simulink model "ESM_TeslaModelS_statKreisfahrt"  (R2020b)
settings: Solver=FixedStepAuto  StartTime=0.0  StopTime=StopTime  FixedStep=SampleTime  RelTol=1e-3
undefined symbols (not defined in the file): ayObs, c_alpha_F, c_alpha_R, c_alpha_rear_mean, DiscIntNeverNeededParam, I_S, init, input_r, m_vehicle, par_TIR, par_VEH, parameter, SelectManeuver, simtime, Single_Track_Model_linear, SingleTrackModel_linear
libraries: pid_lib x5, simulink x3, dspsigops x2, vehicle_model x1
(part 1 of 4)
settings Model: SimulationMode=accelerator  OrderedModelArguments=off  Creator=Johannes  LastModifiedBy=ga69qig
settings DataIOCC: SaveOutput=off  DSMLogging=off  SaveTime=off  ReturnWorkspaceOutputs=off
settings OptimizationCC: EfficientMapNaN2IntZero=off
settings DebuggingCC: ArithmeticOperatorsInVariantConditions=warning
settings HardwareCC: TargetBitPerPointer=64  TargetBitPerSizeT=64  TargetBitPerPtrDiffT=64  TargetLongLongMode=on  TargetIntDivRoundTo=Zero  TargetEndianess=LittleEndian  TargetWordSize=64  TargetHWDeviceType=MATLAB Host  ProdEqTarget=off
settings SFSimCC: SimUseLocalCustomCode=off  CustomCodeUndefinedFunction=UseInterfaceOnly
settings RTWCC: RTWUseLocalCustomCode=off
settings CodeAppCC: MaxIdLength=128
settings GRTTargetCC: TargetLangStandard=C89/C90 (ANSI)  CombineOutputUpdateFcns=off  GRTInterface=on

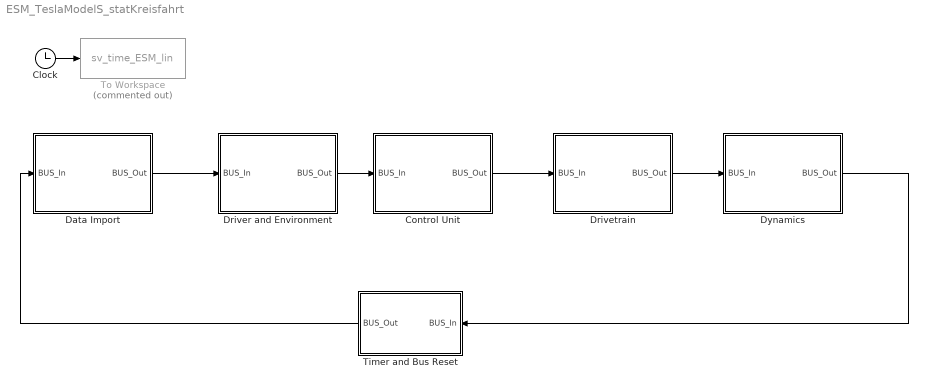
== system ESM_TeslaModelS_statKreisfahrt ==
  Clock : Clock
  Control Unit : Subsystem
      mask help:
      | <Author> Alexander Koch based on Stefan Müller, Stephan Rohr
      | <Date> 03/04/2017
      |
      | <Description>
      | Consist of a Bus In and a Bus Out Block. To Select Signals from the Bus open the Bus In Block, to write signals to the Bus under a certain tab name open the bus out block. For further information, please read the discription of the Bus In and Bus out Block
      |
      | The Block automaticlly disconnects the link to the library block after opening the first time
      |
      | <Parameters>
      | -
      |
      | <Inputs>
      | BUS_In [Bus]
      |
      | <Outputs>
      | Bus_Out [Bus]
      settings: OpenFcn=|
      | set_param(gcb(),'LinkStatus','none')
      | open_system(gcb(),'force')
  Data Import : Subsystem
      mask help:
      | <Author> Alexander Koch based on Stefan Müller, Stephan Rohr
      | <Date> 03/04/2017
      |
      | <Description>
      | Consist of a Bus In and a Bus Out Block. To Select Signals from the Bus open the Bus In Block, to write signals to the Bus under a certain tab name open the bus out block. For further information, please read the discription of the Bus In and Bus out Block
      |
      | The Block automaticlly disconnects the link to the library block after opening the first time
      |
      | <Parameters>
      | -
      |
      | <Inputs>
      | BUS_In [Bus]
      |
      | <Outputs>
      | Bus_Out [Bus]
      settings: OpenFcn=|
      | set_param(gcb(),'LinkStatus','none')
      | open_system(gcb(),'force')
  Driver and Environment : Subsystem
      mask help:
      | <Author> Alexander Koch based on Stefan Müller, Stephan Rohr
      | <Date> 03/04/2017
      |
      | <Description>
      | Consist of a Bus In and a Bus Out Block. To Select Signals from the Bus open the Bus In Block, to write signals to the Bus under a certain tab name open the bus out block. For further information, please read the discription of the Bus In and Bus out Block
      |
      | The Block automaticlly disconnects the link to the library block after opening the first time
      |
      | <Parameters>
      | -
      |
      | <Inputs>
      | BUS_In [Bus]
      |
      | <Outputs>
      | Bus_Out [Bus]
      settings: OpenFcn=|
      | set_param(gcb(),'LinkStatus','none')
      | open_system(gcb(),'force')
  Drivetrain : Subsystem
      mask help:
      | <Author> Alexander Koch based on Stefan Müller, Stephan Rohr
      | <Date> 03/04/2017
      |
      | <Description>
      | Consist of a Bus In and a Bus Out Block. To Select Signals from the Bus open the Bus In Block, to write signals to the Bus under a certain tab name open the bus out block. For further information, please read the discription of the Bus In and Bus out Block
      |
      | The Block automaticlly disconnects the link to the library block after opening the first time
      |
      | <Parameters>
      | -
      |
      | <Inputs>
      | BUS_In [Bus]
      |
      | <Outputs>
      | Bus_Out [Bus]
      settings: OpenFcn=|
      | set_param(gcb(),'LinkStatus','none')
      | open_system(gcb(),'force')
  Dynamics : Subsystem
      mask help:
      | <Author> Alexander Koch based on Stefan Müller, Stephan Rohr
      | <Date> 03/04/2017
      |
      | <Description>
      | Consist of a Bus In and a Bus Out Block. To Select Signals from the Bus open the Bus In Block, to write signals to the Bus under a certain tab name open the bus out block. For further information, please read the discription of the Bus In and Bus out Block
      |
      | The Block automaticlly disconnects the link to the library block after opening the first time
      |
      | <Parameters>
      | -
      |
      | <Inputs>
      | BUS_In [Bus]
      |
      | <Outputs>
      | Bus_Out [Bus]
      settings: OpenFcn=|
      | set_param(gcb(),'LinkStatus','none')
      | open_system(gcb(),'force')
  Timer and Bus Reset : Subsystem
      mask help:
      | <Author> Alexander Koch based on Stefan Müller, Stephan Rohr
      | <Date> 03/04/2017
      |
      | <Description>
      | Initiate a new timestep and creates the Bus_Old with all data of the last time step
      settings: OpenFcn=|
      | set_param(gcb(),'LinkStatus','none')
      | open_system(gcb(),'mask')
      mask DialogControl RefreshBus Prompt: Refresh Bus
      mask DialogControl RefreshBus Callback: TimerandBusResetRefreshBus()
  To Workspace : ToWorkspace  Commented=on  VariableName=sv_time_ESM_lin  SampleTime=-1
      settings: Decimation=savedec  Save2DSignal=2-D array (concatenate along first dimension)
  wires:
  Driver and Environment/1(BUS_Out) -> Control Unit/1(BUS_In)
  Control Unit/1(BUS_Out) -> Drivetrain/1(BUS_In)
  Data Import/1(BUS_Out) -> Driver and Environment/1(BUS_In)
  Drivetrain/1(BUS_Out) -> Dynamics/1(BUS_In)
  Dynamics/1(BUS_Out) -> Timer and Bus Reset/1(BUS_In)
  Timer and Bus Reset/1(BUS_Out) -> Data Import/1(BUS_In)
  Clock/1 -> To Workspace/1

== system ESM_TeslaModelS_statKreisfahrt/Control Unit ==
  BUS_In : Inport
  BUS IN : Subsystem
      mask help:
      | <Author> Alexander Koch, Benedikt Danquah based on Stefan Müller [1], Stephan Rohr [2]  </Author>
      |
      | <Date> 02/05/2017</Date>
      |
      | <Description>
      | Automated BUS IN Block for the Bus System. After the Bus In is connected and receives signals it is possible to choose the required signals by clicking on the block. After choosing the signals it is possible to push the Refresh button. This button builds the required amount of outputs, connects the Bus Selector and the Outputs and rename all the outputs with the corresponding signal name. The Block automaticlly disconnects the link to the library block after opening the first time
      | </Description>
      mask init:
      | BusInInitFct()
      settings: OpenFcn=|
      | set_param(gcb(),'LinkStatus','none')
      | open_system(gcb(),'mask')
      | open_system(strcat(gcb(),'/Bus Selector'),'Parameter')
      mask Help:
      | <Parameters>
      | -
      | </Parameters>
      | 
      | <Inputs>
      | Bus [Bus]
      | </Inputs>
      | 
      | <Outputs>
      | Bus [Bus]
      | SignalName[-]
      | </Outputs>
      | 
      | <Sources>
      | [1] S. Mueller, S. Rohr, W. Schmid, and M. Lienkamp, “Analysing the Influence of Driver Behaviour and Tuning Measures on Battery Aging and Residual Value of Electric Vehicles,” in Proc. EVS30 Symposium, Stuttgart, 2017, pp. 1–12.
      | [2] S. Rohr, “Technisch-wirtschaftliche Analyse des Zweitnutzungs- potentials von Lithium-Ionen-Traktionsbatterien,” Dissertation, Institute of Automotive Technology, Technical University Munich, Munich, 2018.
      | </Sources>
      mask DialogControl Container3 Prompt: Documentation:
      mask DialogControl Control3 Prompt: %<MaskHelp>
      mask DialogControl ParameterGroupVar Prompt: Refresh
      mask DialogControl RefreshOutputs Prompt: Refresh all Output Names
      mask DialogControl RefreshOutputs Callback: BusInInitFct()
  BUS OUT : Subsystem  mask{NumberofInputs=4, NameSys='Control Unit'}
      mask prompts: NumberofInputs "Numper of costum inputs"; NameSys "Name of Bus Subsystem"
      mask help:
      | <Author> Alexander Koch, Benedikt Danquah based on Stefan Müller [1], Stephan Rohr [2]  </Author>
      |
      | <Date> 02/05/2017</Date>
      |
      | <Description>
      | Automated BUS Out Block for the Bus System. Allows to enter the Number of costum inputs and the name of the bus system. After entering the parameters the required amout of Inputs are built and connected to the Bus Creator. The signal names that are connected to the inputs In1, ..., InN are automatically adopted at the Bus signal names and can be found in the Bus under the name of the Bus Subsystem. If the signal (line) to the Inport has no name, the name of the previous blocks outport is taken. If this is not possible, the name if the previous block is taken for the Bus signal name.
      |
      | Additional, there are two buttons. The Refresh Input Names refreshes all Input Names. This is required if signal names are changed or signals are connected for the first time. To build a new system or if another Subsystem is added between existing subsystems, the Refresh Bus Selector is required at every subsystem that is calculated after the new subsystem.
      |
      | The Block automaticlly disconnects the link to the library block after opening the first time
      | </Description>
      mask init:
      | BusRefreshInputs()
      settings: OpenFcn=|
      | set_param(gcb(),'LinkStatus','none')
      | open_system(gcb(),'mask')
      mask Help:
      | <Parameters>
      | Number of costum inputs [-]
      | Name of Bus Subsystem ['abc']
      | </Parameters>
      | 
      | <Inputs>
      | Bus [Bus]
      | In1 [ ]
      | </Inputs>
      | 
      | <Outputs>
      | Bus [Bus]
      | </Outputs>
      | 
      | <Sources>
      | [1] S. Mueller, S. Rohr, W. Schmid, and M. Lienkamp, “Analysing the Influence of Driver Behaviour and Tuning Measures on Battery Aging and Residual Value of Electric Vehicles,” in Proc. EVS30 Symposium, Stuttgart, 2017, pp. 1–12.
      | [2] S. Rohr, “Technisch-wirtschaftliche Analyse des Zweitnutzungs- potentials von Lithium-Ionen-Traktionsbatterien,” Dissertation, Institute of Automotive Technology, Technical University Munich, Munich, 2018.
      | </Sources>
      mask DialogControl Container4 Prompt: Documentation:
      mask DialogControl Control4 Prompt: %<MaskHelp>
      mask DialogControl Container3 Prompt: Refresh
      mask DialogControl RefreshInputNames Prompt: Refresh Input Names
      mask DialogControl RefreshInputNames Callback: BusRefreshLineNames()
      mask DialogControl RefreshBusSelector Prompt: Refresh Bus Selector
      mask DialogControl RefreshBusSelector Callback: BusRefreshBusSelector()
  Control Unit Simple : Subsystem  AncestorBlock=Control_Unit_Simple/Control Unit Simple  mask(SB){Brake_Distribution_Front=0.5, MaxBrkTrq=4200, MaxMotorTrqFront=355.7750901796057, MaxMotorTrqRear=355.7750901796057, LocalSampleTime=-1}
      mask prompts: Brake_Distribution_Front "Brake Distribution Front"; MaxBrkTrq "Maximal Braking Torque"; MaxMotorTrqFront "Maximal Motor Torque Front"; MaxMotorTrqRear "Maximal Motor Torque Rear"; LocalSampleTime "Local System Sample-Time [s]"
      mask help:
      | <Author> Alexander Koch, Benedikt Danquah based on Stefan Müller [1], Stephan Rohr [2]  </Author>
      | <Date> 03/04/2017 </Date>
      |
      | <Description>
      | Requires acceleration pedal position, braking pedal position, a brake distribution, the maximal possible braking torque and tha maximal motor torque and calculates a target drive system torque and a target braking torque for front and rear axle. Minimum drive torques is zero.
      | </Description>
      mask init:
      | GlobalSampleTime = CalcGlobalSampleTime(LocalSampleTime);
      mask Help:
      | <Parameters>
      | Brake distribution front [-]
      | 	<Min> 0 </Min>
      | 	<Max> 1 </Max>
      | Maximal braking torque [Nm]
      | Maximal motor torque [Nm]
      | Local System Sample-Time [s]
      | 	<Min> GlobalSampleTime </Min>
      | Global Sample-Time [s]
      | </Parameters>
      | 
      | <Inputs>
      | AccPedalPos [-]
      | 	<Min> 0 </Min>
      | 	<Max> 1 </Max>
      | BrakePedalPos [-]
      | 	<Min>0 </Min>
      | 	<Max> 1 </Max>
      | </Inputs>
      | 
      | <Outputs>
      | TargetDriveTrqFront [Nm]
      | 	<Min> 0 </Min>
      | TargetDriveTrqRear [Nm]
      | 	<Min> 0 </Min>
      | TargetBrakeTrqFrontAxle [Nm]
      | 	<Max> 0 </Max>
      | TargetBrakeTrqRearAxle [Nm]
      | 	<Max> 0 </Max>
      | </Outputs>
      | <Sources>
      | [1] S. Mueller, S. Rohr, W. Schmid, and M. Lienkamp, “Analysing the Influence of Driver Behaviour and Tuning Measures on Battery Aging and Residual Value of Electric Vehicles,” in Proc. EVS30 Symposium, Stuttgart, 2017, pp. 1–12.
      | [2] S. Rohr, “Technisch-wirtschaftliche Analyse des Zweitnutzungs- potentials von Lithium-Ionen-Traktionsbatterien,” Dissertation, Institute of Automotive Technology, Technical University Munich, Munich, 2018.
      | </Sources>
      mask TypeOptions Brake_Distribution_Front: Brake_Distribution_Front/Value
      mask TypeOptions MaxBrkTrq: MaxBrakeTorque/Value
      mask TypeOptions MaxMotorTrqFront: MaxMotorTorque Front/Value
      mask TypeOptions MaxMotorTrqRear: MaxMotorTorque Rear/Value
      mask TypeOptions LocalSampleTime: AccPedalPos [-]/SampleTime | BrakePedalPos [-]/SampleTime
      mask DialogControl Container3 Prompt: Documentation:
      mask DialogControl DescHelpVar Prompt: %<MaskHelp>
      mask DialogControl Container5 Prompt: Sample Time
      mask Display:
      | [picturexpos,pictureypos,picturewidth,pictureheight] = ...
      |     CalcBlockPicturePosition(gcb,1,0.01,0.1,80,120); % calculating picture position depending on Block size and minimum margin size
      | image('Control_Unit_Simple.svg',[picturexpos pictureypos picturewidth pictureheight]) % plot picture to block
  BUS_Out : Outport
  wires:
  BUS_In/1 -> BUS IN/1(BUS_In)
  BUS OUT/1(BUS_OUT) -> BUS_Out/1
  BUS IN/1(BUS) -> BUS OUT/1(BUS)
  BUS IN/2(AccPedalPos [-]) -> Control Unit Simple/1(AccPedalPos [-])
  BUS IN/3(BrakePedalPos [-]) -> Control Unit Simple/2(BrakePedalPos [-])
  Control Unit Simple/3(TargetBrakeTrqFrontAxle [Nm]) -> BUS OUT/4(In3)  "TargetBrakeTrqFrontAxle [Nm]"
  Control Unit Simple/4(TargetBrakeTrqRearAxle [Nm]) -> BUS OUT/5(In4)  "TargetBrakeTrqRearAxle [Nm]"
  Control Unit Simple/2("TargetDriveTrqRear [Nm] ") -> BUS OUT/3(In2)  "TargetDriveTrqRear [Nm]"
  Control Unit Simple/1("TargetDriveTrqFront [Nm] ") -> BUS OUT/2(In1)  "TargetDriveTrqFront [Nm]"

== system ESM_TeslaModelS_statKreisfahrt/Data Import ==
  BUS_In : Inport
  BUS IN : Subsystem
      mask help:
      | <Author> Alexander Koch based on Stefan Müller, Stephan Rohr
      | <Date> 02/05/2017
      |
      | <Description>
      | Automated BUS IN Block for the Bus System. After the Bus In is connected and receives signals it is possible to choose the required signals by clicking on the block. After choosing the signals it is possible to push the Refresh button. This button builds the required amount of outputs, connects the Bus Selector and the Outputs and rename all the outputs with the corresponding signal name.
      |
      | The Block automaticlly disconnects the link to the library block after opening the first time
      |
      | <Parameters>
      | -
      |
      | <Inputs>
      | Bus [Bus]
      |
      | <Outputs>
      | Bus [Bus]
      | SignalName[-]
      mask init:
      | BusInInitFct()
      settings: OpenFcn=|
      | set_param(gcb(),'LinkStatus','none')
      | open_system(gcb(),'mask')
      | open_system(strcat(gcb(),'/Bus Selector'),'Parameter')
      mask DialogControl ParameterGroupVar Prompt: Refresh
      mask DialogControl RefreshOutputs Prompt: Refresh all Output Names
      mask DialogControl RefreshOutputs Callback: BusInInitFct()
  BUS OUT : Subsystem  mask{NumberofInputs=3, NameSys='Data Import'}
      mask prompts: NumberofInputs "Numper of costum inputs"; NameSys "Name of Bus Subsystem"
      mask help:
      | <Author> Alexander Koch based on Stefan Müller, Stephan Rohr
      | <Date> 02/05/2017
      |
      | <Description>
      | Automated BUS Out Block for the Bus System. Allows to enter the Number of costum inputs and the name of the bus system. After entering the parameters the required amout of Inputs are built and connected to the Bus Creator. The signal names that are connected to the inputs In1, ..., InN are automatically adopted at the Bus signal names and can be found in the Bus under the name of the Bus Subsystem. If the signal (line) to the Inport has no name, the name of the previous blocks outport is taken. If this is not possible, the name if the previous block is taken for the Bus signal name.
      |
      | Additional, there are two buttons. The Refresh Input Names refreshes all Input Names. This is required if signal names are changed or signals are connected for the first time. To build a new system or if another Subsystem is added between existing subsystems, the Refresh Bus Selector is required at every subsystem that is calculated after the new subsystem.
      |
      | The Block automaticlly disconnects the link to the library block after opening the first time
      |
      | <Parameters>
      | Number of costum inputs [-]
      | Name of Bus Subsystem ['abc']
      |
      | <Inputs>
      | Bus [Bus]
      | In1 [ ]
      |
      | <Outputs>
      | Bus [Bus]
      mask init:
      | BusRefreshInputs()
      settings: OpenFcn=|
      | set_param(gcb(),'LinkStatus','none')
      | open_system(gcb(),'mask')
      mask DialogControl Container3 Prompt: Refresh
      mask DialogControl RefreshInputNames Prompt: Refresh Input Names
      mask DialogControl RefreshInputNames Callback: BusRefreshLineNames()
      mask DialogControl RefreshBusSelector Prompt: Refresh Bus Selector
      mask DialogControl RefreshBusSelector Callback: BusRefreshBusSelector()
  Constant : Constant  Value=input_r
  From Workspace1 : FromWorkspace  VariableName=v_maneuver
  From Workspace2 : FromWorkspace  VariableName=delta_maneuver
  Gain : Gain  Gain=pi/180
  Terminator : Terminator
  BUS_Out : Outport  VectorParamsAs1DForOutWhenUnconnected=off
  wires:
  BUS_In/1 -> BUS IN/1(BUS_In)
  BUS OUT/1(BUS_OUT) -> BUS_Out/1
  BUS IN/1(BUS) -> BUS OUT/1(BUS)
  BUS IN/2(omega_F [rad/s]) -> Terminator/1
  From Workspace1/1 -> BUS OUT/3(In2)  "Traget_Velocity [m/s]"
  Gain/1 -> BUS OUT/4(In3)  "Target_Steering_Angle [rad]"
  From Workspace2/1 -> Gain/1  "Target_Steering_Angle [Grad]"
  Constant/1 -> BUS OUT/2(In1)  "Target_Radius [m]"

== system ESM_TeslaModelS_statKreisfahrt/Driver and Environment ==
  BUS_In : Inport
  BUS IN : Subsystem
      mask help:
      | <Author> Alexander Koch based on Stefan Müller, Stephan Rohr
      | <Date> 02/05/2017
      |
      | <Description>
      | Automated BUS IN Block for the Bus System. After the Bus In is connected and receives signals it is possible to choose the required signals by clicking on the block. After choosing the signals it is possible to push the Refresh button. This button builds the required amount of outputs, connects the Bus Selector and the Outputs and rename all the outputs with the corresponding signal name.
      |
      | The Block automaticlly disconnects the link to the library block after opening the first time
      |
      | <Parameters>
      | -
      |
      | <Inputs>
      | Bus [Bus]
      |
      | <Outputs>
      | Bus [Bus]
      | SignalName[-]
      mask init:
      | BusInInitFct()
      settings: OpenFcn=|
      | set_param(gcb(),'LinkStatus','none')
      | open_system(gcb(),'mask')
      | open_system(strcat(gcb(),'/Bus Selector'),'Parameter')
      mask DialogControl ParameterGroupVar Prompt: Refresh
      mask DialogControl RefreshOutputs Prompt: Refresh all Output Names
      mask DialogControl RefreshOutputs Callback: BusInInitFct()
  BUS OUT : Subsystem  mask{NumberofInputs=3, NameSys='Driver and Environment'}
      mask prompts: NumberofInputs "Numper of costum inputs"; NameSys "Name of Bus Subsystem"
      mask help:
      | <Author> Alexander Koch based on Stefan Müller, Stephan Rohr
      | <Date> 02/05/2017
      |
      | <Description>
      | Automated BUS Out Block for the Bus System. Allows to enter the Number of costum inputs and the name of the bus system. After entering the parameters the required amout of Inputs are built and connected to the Bus Creator. The signal names that are connected to the inputs In1, ..., InN are automatically adopted at the Bus signal names and can be found in the Bus under the name of the Bus Subsystem. If the signal (line) to the Inport has no name, the name of the previous blocks outport is taken. If this is not possible, the name if the previous block is taken for the Bus signal name.
      |
      | Additional, there are two buttons. The Refresh Input Names refreshes all Input Names. This is required if signal names are changed or signals are connected for the first time. To build a new system or if another Subsystem is added between existing subsystems, the Refresh Bus Selector is required at every subsystem that is calculated after the new subsystem.
      |
      | The Block automaticlly disconnects the link to the library block after opening the first time
      |
      | <Parameters>
      | Number of costum inputs [-]
      | Name of Bus Subsystem ['abc']
      |
      | <Inputs>
      | Bus [Bus]
      | In1 [ ]
      |
      | <Outputs>
      | Bus [Bus]
      mask init:
      | BusRefreshInputs()
      settings: OpenFcn=|
      | set_param(gcb(),'LinkStatus','none')
      | open_system(gcb(),'mask')
      mask DialogControl Container3 Prompt: Refresh
      mask DialogControl RefreshInputNames Prompt: Refresh Input Names
      mask DialogControl RefreshInputNames Callback: BusRefreshLineNames()
      mask DialogControl RefreshBusSelector Prompt: Refresh Bus Selector
      mask DialogControl RefreshBusSelector Callback: BusRefreshBusSelector()
  Lenkradwinkelsprung : Subsystem  TreatAsAtomicUnit=on
  Multiport Switch : MultiPortSwitch  Inputs=5
  Multiport Switch1 : MultiPortSwitch  Inputs=5
  Multiport Switch2 : MultiPortSwitch  Inputs=5
  SelectManeuver : Constant  Value=SelectManeuver
  Sinuslenken : Subsystem  TreatAsAtomicUnit=on
  quasistationare Kreisfahrt : Subsystem  TreatAsAtomicUnit=on
  quasistationare Kreisfahrt mit Lastwechsel Beschleunigung : Subsystem  TreatAsAtomicUnit=on
  quasistationare Kreisfahrt mit Lastwechsel Verzogerung : Subsystem  TreatAsAtomicUnit=on
  BUS_Out : Outport  VectorParamsAs1DForOutWhenUnconnected=off
  wires:
  BUS OUT/1(BUS_OUT) -> BUS_Out/1
  BUS_In/1 -> BUS IN/1(BUS_In)
  Lenkradwinkelsprung/3(BrakePedalPos [-]) -> Multiport Switch2/5
  quasistationare Kreisfahrt/1(delta_h) -> Multiport Switch/2
  BUS IN/7(Target_Steering_Angle [rad]) -> Sinuslenken/3(Target_Steering_Angle [rad])
  Multiport Switch1/1 -> BUS OUT/3(In2)  "AccPedalPos [-]"
  quasistationare Kreisfahrt mit Lastwechsel Verzogerung/3(BrakePedalPos [-]) -> Multiport Switch2/3
  quasistationare Kreisfahrt mit Lastwechsel Verzogerung/1(delta_h) -> Multiport Switch/3  "delta_h"
  Sinuslenken/2(AccPedalPos [-]) -> Multiport Switch1/6
  Sinuslenken/1(delta_h) -> Multiport Switch/6
  BUS IN/3(Traget_Velocity [m/s]) -> quasistationare Kreisfahrt mit Lastwechsel Verzogerung/2(TargetVelocity [m/s]), quasistationare Kreisfahrt mit Lastwechsel Beschleunigung/2(TargetVelocity [m/s]), Lenkradwinkelsprung/2(TargetVelocity [m/s]), Sinuslenken/2(TargetVelocity [m/s]), quasistationare Kreisfahrt/2(TargetVelocity [m/s])
  BUS IN/6(vx [m/s]) -> quasistationare Kreisfahrt mit Lastwechsel Beschleunigung/5(VelocityX [m/s]), quasistationare Kreisfahrt mit Lastwechsel Verzogerung/5(VelocityX [m/s]), quasistationare Kreisfahrt/5(VelocityX [m/s])
  quasistationare Kreisfahrt mit Lastwechsel Verzogerung/2(AccPedalPos [-]) -> Multiport Switch1/3
  quasistationare Kreisfahrt/2(AccPedalPos [-]) -> Multiport Switch1/2
  quasistationare Kreisfahrt/3(BrakePedalPos [-]) -> Multiport Switch2/2
  BUS IN/5(Target_Radius [m]) -> quasistationare Kreisfahrt mit Lastwechsel Beschleunigung/4(TargetRadius [m]), quasistationare Kreisfahrt mit Lastwechsel Verzogerung/4(TargetRadius [m]), quasistationare Kreisfahrt/4(TargetRadius [m])
  Multiport Switch2/1 -> BUS OUT/4(In3)  "BrakePedalPos [-]"
  Lenkradwinkelsprung/1(delta_h) -> Multiport Switch/5
  BUS IN/1(BUS) -> BUS OUT/1(BUS)
  Multiport Switch/1 -> BUS OUT/2(In1)  "delta_h"
  BUS IN/4(ay [m/s^2]) -> quasistationare Kreisfahrt mit Lastwechsel Verzogerung/3(AccelerationY [m/s]), quasistationare Kreisfahrt mit Lastwechsel Beschleunigung/3(AccelerationY [m/s]), quasistationare Kreisfahrt/3(AccelerationY [m/s])
  Sinuslenken/3(BrakePedalPos [-]) -> Multiport Switch2/6
  SelectManeuver/1 -> Multiport Switch/1, Multiport Switch2/1, Multiport Switch1/1
  BUS IN/2(v) -> quasistationare Kreisfahrt mit Lastwechsel Verzogerung/1(Velocity [m/s]), quasistationare Kreisfahrt mit Lastwechsel Beschleunigung/1(Velocity [m/s]), Lenkradwinkelsprung/1(Velocity [m/s]), Sinuslenken/1(Velocity [m/s]), quasistationare Kreisfahrt/1(Velocity [m/s])
  Lenkradwinkelsprung/2(AccPedalPos [-]) -> Multiport Switch1/5
  quasistationare Kreisfahrt mit Lastwechsel Beschleunigung/1(delta_h) -> Multiport Switch/4
  quasistationare Kreisfahrt mit Lastwechsel Beschleunigung/2(AccPedalPos [-]) -> Multiport Switch1/4
  quasistationare Kreisfahrt mit Lastwechsel Beschleunigung/3(BrakePedalPos [-]) -> Multiport Switch2/4

== system ESM_TeslaModelS_statKreisfahrt/Drivetrain ==
  BUS_In : Inport
  Axle Drive Front : Subsystem  AncestorBlock=Axle_Drive/Axle Drive  mask(SB){ratio=9.34, trq_eff=0.9684, LocalSampleTime=-1}
      mask prompts: ratio "Ratio [-]"; trq_eff "Efficiency [-]"; LocalSampleTime "Local System Sample-Time [s]"
      mask help:
      | <Author> Jan Breithaupt </Author>
      | <Date> 05/03/2018 </Date>
      | <Predecessor> Michael Fries </Predecessor>
      |
      | <Description>
      | Calculates torque, rotational speed and moment of inertia acording to the ratio of the axle drive.
      | </Description>
      mask init:
      | GlobalSampleTime = CalcGlobalSampleTime(LocalSampleTime);
      mask Help:
      | <Parameters>
      | Ratio [-]
      | Efficiency [-]
      | Local System Sample-Time [s]
      | 	<Min> GlobalSampleTime </Min>
      | Global Sample-Time [s]
      | </Parameters>
      | 
      | <Inputs>
      | RotSpdWheel [rad/s]
      | GearboxEntranceTrq [Nm]
      | JredIn [kg m^2]
      | </Inputs>
      | 
      | <Outputs>
      | RotSpdGearboxOut [rad/s]
      | WheelMotTrq[Nm]
      | JredOut [kg m^2]
      | </Outputs>
      mask TypeOptions LocalSampleTime: GearboxEntranceTorque [Nm]/SampleTime | RotSpdWheel [rad//s]/SampleTime | JredIn [kg//m^2]/SampleTime
      mask DialogControl Container3 Prompt: Documentation:
      mask DialogControl Control2 Prompt: %<MaskHelp>
      mask DialogControl Container5 Prompt: Sample Time
      mask Display:
      | [picturexpos,pictureypos,picturewidth,pictureheight] = ...
      |     CalcBlockPicturePosition(gcb,1,0.01,0.1,100,100); % calculating picture position depending on Block size and minimum margin size
      | image('Axle_Drive.svg',[picturexpos pictureypos picturewidth pictureheight]); % plot picture to block
  Axle Drive Rear : Subsystem  AncestorBlock=Axle_Drive/Axle Drive  mask(SB){ratio=9.34, trq_eff=0.9684, LocalSampleTime=-1}
      mask prompts: ratio "Ratio [-]"; trq_eff "Efficiency [-]"; LocalSampleTime "Local System Sample-Time [s]"
      mask help:
      | <Author> Jan Breithaupt </Author>
      | <Date> 05/03/2018 </Date>
      | <Predecessor> Michael Fries </Predecessor>
      |
      | <Description>
      | Calculates torque, rotational speed and moment of inertia acording to the ratio of the axle drive.
      | </Description>
      mask init:
      | GlobalSampleTime = CalcGlobalSampleTime(LocalSampleTime);
      mask Help:
      | <Parameters>
      | Ratio [-]
      | Efficiency [-]
      | Local System Sample-Time [s]
      | 	<Min> GlobalSampleTime </Min>
      | Global Sample-Time [s]
      | </Parameters>
      | 
      | <Inputs>
      | RotSpdWheel [rad/s]
      | GearboxEntranceTrq [Nm]
      | JredIn [kg m^2]
      | </Inputs>
      | 
      | <Outputs>
      | RotSpdGearboxOut [rad/s]
      | WheelMotTrq[Nm]
      | JredOut [kg m^2]
      | </Outputs>
      mask TypeOptions LocalSampleTime: GearboxEntranceTorque [Nm]/SampleTime | RotSpdWheel [rad//s]/SampleTime | JredIn [kg//m^2]/SampleTime
      mask DialogControl Container3 Prompt: Documentation:
      mask DialogControl Control2 Prompt: %<MaskHelp>
      mask DialogControl Container5 Prompt: Sample Time
      mask Display:
      | [picturexpos,pictureypos,picturewidth,pictureheight] = ...
      |     CalcBlockPicturePosition(gcb,1,0.01,0.1,100,100); % calculating picture position depending on Block size and minimum margin size
      | image('Axle_Drive.svg',[picturexpos pictureypos picturewidth pictureheight]); % plot picture to block
  BUS IN : Subsystem
      mask help:
      | <Author> Alexander Koch, Benedikt Danquah based on Stefan Müller [1], Stephan Rohr [2]  </Author>
      |
      | <Date> 02/05/2017</Date>
      |
      | <Description>
      | Automated BUS IN Block for the Bus System. After the Bus In is connected and receives signals it is possible to choose the required signals by clicking on the block. After choosing the signals it is possible to push the Refresh button. This button builds the required amount of outputs, connects the Bus Selector and the Outputs and rename all the outputs with the corresponding signal name. The Block automaticlly disconnects the link to the library block after opening the first time
      | </Description>
      mask init:
      | BusInInitFct()
      settings: OpenFcn=|
      | set_param(gcb(),'LinkStatus','none')
      | open_system(gcb(),'mask')
      | open_system(strcat(gcb(),'/Bus Selector'),'Parameter')
      mask Help:
      | <Parameters>
      | -
      | </Parameters>
      | 
      | <Inputs>
      | Bus [Bus]
      | </Inputs>
      | 
      | <Outputs>
      | Bus [Bus]
      | SignalName[-]
      | </Outputs>
      | 
      | <Sources>
      | [1] S. Mueller, S. Rohr, W. Schmid, and M. Lienkamp, “Analysing the Influence of Driver Behaviour and Tuning Measures on Battery Aging and Residual Value of Electric Vehicles,” in Proc. EVS30 Symposium, Stuttgart, 2017, pp. 1–12.
      | [2] S. Rohr, “Technisch-wirtschaftliche Analyse des Zweitnutzungs- potentials von Lithium-Ionen-Traktionsbatterien,” Dissertation, Institute of Automotive Technology, Technical University Munich, Munich, 2018.
      | </Sources>
      mask DialogControl Container3 Prompt: Documentation:
      mask DialogControl Control3 Prompt: %<MaskHelp>
      mask DialogControl ParameterGroupVar Prompt: Refresh
      mask DialogControl RefreshOutputs Prompt: Refresh all Output Names
      mask DialogControl RefreshOutputs Callback: BusInInitFct()
  BUS OUT : Subsystem  mask{NumberofInputs=4, NameSys='Drivetrain'}
      mask prompts: NumberofInputs "Numper of costum inputs"; NameSys "Name of Bus Subsystem"
      mask help:
      | <Author> Alexander Koch, Benedikt Danquah based on Stefan Müller [1], Stephan Rohr [2]  </Author>
      |
      | <Date> 02/05/2017</Date>
      |
      | <Description>
      | Automated BUS Out Block for the Bus System. Allows to enter the Number of costum inputs and the name of the bus system. After entering the parameters the required amout of Inputs are built and connected to the Bus Creator. The signal names that are connected to the inputs In1, ..., InN are automatically adopted at the Bus signal names and can be found in the Bus under the name of the Bus Subsystem. If the signal (line) to the Inport has no name, the name of the previous blocks outport is taken. If this is not possible, the name if the previous block is taken for the Bus signal name.
      |
      | Additional, there are two buttons. The Refresh Input Names refreshes all Input Names. This is required if signal names are changed or signals are connected for the first time. To build a new system or if another Subsystem is added between existing subsystems, the Refresh Bus Selector is required at every subsystem that is calculated after the new subsystem.
      |
      | The Block automaticlly disconnects the link to the library block after opening the first time
      | </Description>
      mask init:
      | BusRefreshInputs()
      settings: OpenFcn=|
      | set_param(gcb(),'LinkStatus','none')
      | open_system(gcb(),'mask')
      mask Help:
      | <Parameters>
      | Number of costum inputs [-]
      | Name of Bus Subsystem ['abc']
      | </Parameters>
      | 
      | <Inputs>
      | Bus [Bus]
      | In1 [ ]
      | </Inputs>
      | 
      | <Outputs>
      | Bus [Bus]
      | </Outputs>
      | 
      | <Sources>
      | [1] S. Mueller, S. Rohr, W. Schmid, and M. Lienkamp, “Analysing the Influence of Driver Behaviour and Tuning Measures on Battery Aging and Residual Value of Electric Vehicles,” in Proc. EVS30 Symposium, Stuttgart, 2017, pp. 1–12.
      | [2] S. Rohr, “Technisch-wirtschaftliche Analyse des Zweitnutzungs- potentials von Lithium-Ionen-Traktionsbatterien,” Dissertation, Institute of Automotive Technology, Technical University Munich, Munich, 2018.
      | </Sources>
      mask DialogControl Container4 Prompt: Documentation:
      mask DialogControl Control4 Prompt: %<MaskHelp>
      mask DialogControl Container3 Prompt: Refresh
      mask DialogControl RefreshInputNames Prompt: Refresh Input Names
      mask DialogControl RefreshInputNames Callback: BusRefreshLineNames()
      mask DialogControl RefreshBusSelector Prompt: Refresh Bus Selector
      mask DialogControl RefreshBusSelector Callback: BusRefreshBusSelector()
  Torque_Berechnung Front : Subsystem  Priority=3  AncestorBlock=ICE_scaling_simple/ICE scaling simple  mask(SB){}
      mask help:
      | <Author> Jan Breithaupt
      | <Date> 05/03/2018
      | <Predecessor> Maximilian Tschochner
      |
      | <Description>
      | Calculates consumption map, inertia und maximum torque of the engine.
      |
      | <Parameters>
      | Engine Type ['abc']
      | Peak power [kW]
      |
      | <Inputs>
      | n [rad/s]
      | v [m/s]
      | TargetTrq [Nm]
      | ICE on [-]
      |
      | <Outputs>
      | OutputTrq[Nm]
      | MomentofIntertia[kg m^2]
      mask DialogControl Container2 Prompt: Parameters
      mask DialogControl get_variables Prompt: show current variables in workspace
      mask DialogControl get_variables Callback: [variables_current_block]=get_current_workspace_parameter();
  Torque_Berechnung Rear : Subsystem  Priority=3  AncestorBlock=ICE_scaling_simple/ICE scaling simple  mask(SB){}
      mask help:
      | <Author> Jan Breithaupt
      | <Date> 05/03/2018
      | <Predecessor> Maximilian Tschochner
      |
      | <Description>
      | Calculates consumption map, inertia und maximum torque of the engine.
      |
      | <Parameters>
      | Engine Type ['abc']
      | Peak power [kW]
      |
      | <Inputs>
      | n [rad/s]
      | v [m/s]
      | TargetTrq [Nm]
      | ICE on [-]
      |
      | <Outputs>
      | OutputTrq[Nm]
      | MomentofIntertia[kg m^2]
      mask DialogControl Container2 Prompt: Parameters
      mask DialogControl get_variables Prompt: show current variables in workspace
      mask DialogControl get_variables Callback: [variables_current_block]=get_current_workspace_parameter();
  BUS_Out : Outport
  wires:
  BUS IN/1(BUS) -> BUS OUT/1(BUS)
  BUS OUT/1(BUS_OUT) -> BUS_Out/1
  BUS_In/1 -> BUS IN/1(BUS_In)
  BUS IN/3(omega_F [rad/s]) -> Axle Drive Front/2(RotSpdWheel [rad/s])
  BUS IN/2(TargetDriveTrqFront [Nm]) -> Torque_Berechnung Front/2(TargetTrq [Nm])
  Torque_Berechnung Front/1(OutputTrq [Nm]) -> Axle Drive Front/1(GearboxEntranceTorque [Nm])
  Axle Drive Front/3(RotSpdGearboxOut [rad/s]) -> Torque_Berechnung Front/1(RotSpd [rad/s])
  Torque_Berechnung Front/2(MomentofInertia [kg m^2]) -> Axle Drive Front/3(JredIn [kg/m^2])
  Torque_Berechnung Rear/1(OutputTrq [Nm]) -> Axle Drive Rear/1(GearboxEntranceTorque [Nm])
  Torque_Berechnung Rear/2(MomentofInertia [kg m^2]) -> Axle Drive Rear/3(JredIn [kg/m^2])
  Axle Drive Rear/3(RotSpdGearboxOut [rad/s]) -> Torque_Berechnung Rear/1(RotSpd [rad/s])
  Axle Drive Front/1(WheelMotTrq [Nm]) -> BUS OUT/2(In1)  "WheelMotTrqFront [Nm]"
  Axle Drive Front/2(JredOut [kg/m^2]) -> BUS OUT/3(In2)  "JredOutFront [kg/m^2]"
  Axle Drive Rear/1(WheelMotTrq [Nm]) -> BUS OUT/4(In3)  "WheelMotTrqRear [Nm]"
  Axle Drive Rear/2(JredOut [kg/m^2]) -> BUS OUT/5(In4)  "JredOutRear [kg/m^2]"
  BUS IN/4(TargetDriveTrqRear [Nm]) -> Torque_Berechnung Rear/2(TargetTrq [Nm])
  BUS IN/5(omega_R [rad/s]) -> Axle Drive Rear/2(RotSpdWheel [rad/s])

== system ESM_TeslaModelS_statKreisfahrt/Dynamics ==
  BUS_In : Inport
  BUS IN : Subsystem
      mask help:
      | <Author> Alexander Koch based on Stefan Müller, Stephan Rohr
      | <Date> 02/05/2017
      |
      | <Description>
      | Automated BUS IN Block for the Bus System. After the Bus In is connected and receives signals it is possible to choose the required signals by clicking on the block. After choosing the signals it is possible to push the Refresh button. This button builds the required amount of outputs, connects the Bus Selector and the Outputs and rename all the outputs with the corresponding signal name.
      |
      | The Block automaticlly disconnects the link to the library block after opening the first time
      |
      | <Parameters>
      | -
      |
      | <Inputs>
      | Bus [Bus]
      |
      | <Outputs>
      | Bus [Bus]
      | SignalName[-]
      mask init:
      | BusInInitFct()
      settings: OpenFcn=|
      | set_param(gcb(),'LinkStatus','none')
      | open_system(gcb(),'mask')
      | open_system(strcat(gcb(),'/Bus Selector'),'Parameter')
      mask DialogControl ParameterGroupVar Prompt: Refresh
      mask DialogControl RefreshOutputs Prompt: Refresh all Output Names
      mask DialogControl RefreshOutputs Callback: BusInInitFct()
  BUS OUT : Subsystem  mask{NumberofInputs=11, NameSys='Dynamics'}
      mask prompts: NumberofInputs "Numper of costum inputs"; NameSys "Name of Bus Subsystem"
      mask help:
      | <Author> Alexander Koch based on Stefan Müller, Stephan Rohr
      | <Date> 02/05/2017
      |
      | <Description>
      | Automated BUS Out Block for the Bus System. Allows to enter the Number of costum inputs and the name of the bus system. After entering the parameters the required amout of Inputs are built and connected to the Bus Creator. The signal names that are connected to the inputs In1, ..., InN are automatically adopted at the Bus signal names and can be found in the Bus under the name of the Bus Subsystem. If the signal (line) to the Inport has no name, the name of the previous blocks outport is taken. If this is not possible, the name if the previous block is taken for the Bus signal name.
      |
      | Additional, there are two buttons. The Refresh Input Names refreshes all Input Names. This is required if signal names are changed or signals are connected for the first time. To build a new system or if another Subsystem is added between existing subsystems, the Refresh Bus Selector is required at every subsystem that is calculated after the new subsystem.
      |
      | The Block automaticlly disconnects the link to the library block after opening the first time
      |
      | <Parameters>
      | Number of costum inputs [-]
      | Name of Bus Subsystem ['abc']
      |
      | <Inputs>
      | Bus [Bus]
      | In1 [ ]
      |
      | <Outputs>
      | Bus [Bus]
      mask init:
      | BusRefreshInputs()
      settings: OpenFcn=|
      | set_param(gcb(),'LinkStatus','none')
      | open_system(gcb(),'mask')
      mask DialogControl Container3 Prompt: Refresh
      mask DialogControl RefreshInputNames Prompt: Refresh Input Names
      mask DialogControl RefreshInputNames Callback: BusRefreshLineNames()
      mask DialogControl RefreshBusSelector Prompt: Refresh Bus Selector
      mask DialogControl RefreshBusSelector Callback: BusRefreshBusSelector()
  Bus Selector : BusSelector  OutputSignals=delta_RF
  Constant : Constant  Value=ayObs
  Constant1 : Constant  Value=0
  Constant2 : Constant  Value=0
  Constant3 : Constant  Value=0
  Constant4 : Constant  Value=m_vehicle
  Constant5 : Constant  Value=c_alpha_F
  Constant6 : Constant  Value=c_alpha_R
  Lenkübersetzung1 : Subsystem
  SingleTrackModel_linear : Subsystem  AncestorBlock=Single_Track_Model_linear/SingleTrackModel_linear  mask(SB){RohAir=1.2041, VEH_m=m_vehicle, VEH_Iz=4.148093318499145e+03, VEH_xSP=1.426000000000000, VEH_g=9.81, VEH_cz=0, VEH_cx=0.561600000000000, VEH_cy=0, VEH_Afront=1, VEH_xDP=1.426000000000000, VEH_yDP=0, VEH_l=2.96, INIT_x=0, INIT_y=0, INIT_psi=parameter.psip0, psip0=parameter.psip0, INIT_zroad_RF0=0, INIT_zroad_LF0=0, INIT_zroad_RR0=0, INIT_zroad_LR0=0, v0=parameter.v0, unloadedRadius_F=0.313977, c_alpha_F=c_alpha_F, unloadedRadius_R=0.313977, c_alpha_R=c_alpha_R}
      mask prompts: RohAir "Air Density [kg/m^3]"; VEH_m "Mass Vehicle [kg]"; VEH_Iz "Inertia of Vehicle about z [kg m^2]"; VEH_xSP "Center of Gravity of Vehicle in x [m]"; VEH_g "Gravity [N/kg]"; VEH_cz "cw-Value in z [-]"; VEH_cx "cw-Value in x [-]"; VEH_cy "cw-Value in y [-]"; VEH_Afront "Front Surface area [m^2]"; VEH_xDP "Pressure point position in x-direction [m]"; VEH_yDP "Pressure point position in y-direction [m]"; VEH_l "Wheel Base [m]"; INIT_x "Initial Position x"; INIT_y "Initial Position y"; INIT_psi "Initial Position psi"; psip0 "Initial psip"; INIT_zroad_RF0 "Initial Road Position z Right Front"; INIT_zroad_LF0 "Initial Road Position z Left Front"; INIT_zroad_RR0 "Initial Road Position z Right Rear"; INIT_zroad_LR0 "Initial Road Position z Left Rear"; v0 "Initial Speed [m/s]"; unloadedRadius_F "Unloaded Radius Front Tire"; c_alpha_F "Lateral Stiffness Front"; unloadedRadius_R "Unloaded Radius Rear Tire"; c_alpha_R "Lateral Stiffness Rear"
      mask help:
      | <Author> Johannes Rühm
      | <Date> 05/12/2018
      |
      | <Description>
      | Single Track Model using a linear tire model. Structure is based on double track model of "Schultze". Lateral Stiffnesses of tires must be calculated with double track model.
      |
      | <Parameters>
      | ...
      |
      | <Inputs>
      | TorqueFront [Nm]
      | TorqueRear [Nm]
      | BrakingTorqueFront [Nm]
      | BrakingTorqueRear [Nm]
      | SteeringAngleFront [rad]
      | zRoadFront [m]
      | zRoadRear [m]
      | VelocityWindX [m/s]
      | VelocityWindY [m/s]
      | VelocityWindZ [m/s]
      | Reset
      |
      | <Outputs>
      | WheelRotation/Velocity [Bus]
      | WheelForces [Bus]
      | WheelMoments [Bus]
      | DynamicWheelRadii [Bus]
      | StaticWheelRadii [Bus]
      | RotaionalAnglesandDerivatives [Bus]
      | x,y,zPositionCenterofGravityandDerivates [Bus]
      | SlipAnglesWheels [Bus]
      | SideSlipAngleandDerivate [Bus]
      | TotalSteeringAngle [Bus]
      | AreodynamicPowerLosses [Bus]
      mask init:
      | %savedec=0;
      | [par_VEH, par_TIR] =  Init_ESM_linear (RohAir,VEH_m,VEH_xSP,VEH_g,VEH_cz,VEH_cx,VEH_cy,VEH_xDP,VEH_yDP,VEH_Iz,VEH_l,VEH_Afront, unloadedRadius_F, c_alpha_F, unloadedRadius_R, c_alpha_R)
      mask DialogControl Container12 Prompt: Vehicle
      mask DialogControl Container13 Prompt: Mass Data
      mask DialogControl Container15 Prompt: Aerodynamics
      mask DialogControl Container18 Prompt: Dimensions
      mask DialogControl Container32 Prompt: Initial Parameters
      mask DialogControl Container4 Prompt: Tire
      mask DialogControl Container6 Prompt: Front
      mask DialogControl Container8 Prompt: Rear
  Terminator : Terminator
  BUS_Out : Outport  VectorParamsAs1DForOutWhenUnconnected=off
  wires:
  BUS_In/1 -> BUS IN/1(BUS_In)
  BUS OUT/1(BUS_OUT) -> BUS_Out/1
  BUS IN/1(BUS) -> BUS OUT/1(BUS)
  Constant1/1 -> SingleTrackModel_linear/6(zRoadFront [m]), SingleTrackModel_linear/7(zRoadRear [m])
  Constant2/1 -> SingleTrackModel_linear/11(Reset)
  Constant3/1 -> SingleTrackModel_linear/8(VelocityWindX [m/s]), SingleTrackModel_linear/9(VelocityWindY [m/s]), SingleTrackModel_linear/10(VelocityWindZ [m/s])
  SingleTrackModel_linear/1(WheelRotation/Velocity [Bus]) -> BUS OUT/2(In1)
  SingleTrackModel_linear/2(WheelForces [Bus]) -> BUS OUT/3(In2)
  SingleTrackModel_linear/3(WheelMoments [Bus]) -> BUS OUT/4(In3)
  SingleTrackModel_linear/4(DynamicWheelRadii [Bus]) -> BUS OUT/5(In4)
  SingleTrackModel_linear/5(StaticWheelRadii [Bus]) -> BUS OUT/6(In5)
  SingleTrackModel_linear/6(RotationalAnglesandDerivates [Bus]) -> BUS OUT/7(In6)
  SingleTrackModel_linear/7(x,y,zPositionCenterofGravityandDerivates [Bus]) -> BUS OUT/8(In7)
  SingleTrackModel_linear/8(SlipAnglesWheels [Bus]) -> BUS OUT/9(In8)
  SingleTrackModel_linear/9(SideSlipAngleandDerivate [Bus]) -> BUS OUT/10(In9)
  SingleTrackModel_linear/11(AreodynamicPowerLosses [Bus]) -> BUS OUT/12(In11)
  SingleTrackModel_linear/10(TotalSteeringAngle [Bus]) -> BUS OUT/11(In10)
  BUS IN/2(WheelMotTrqFront [Nm]) -> SingleTrackModel_linear/1(TorqueFront [Nm])
  BUS IN/3(WheelMotTrqRear [Nm]) -> SingleTrackModel_linear/2(TorqueRear [Nm])
  BUS IN/4(TargetBrakeTrqFrontAxle [Nm]) -> SingleTrackModel_linear/3(BrakingTorqueFront [Nm])
  BUS IN/5(TargetBrakeTrqRearAxle [Nm]) -> SingleTrackModel_linear/4(BrakingTorqueRear [Nm])
  Constant/1 -> Terminator/1  "ayObs"
  Constant4/1 -> SingleTrackModel_linear/12(m_vehicle)
  Constant5/1 -> SingleTrackModel_linear/13(c_alpha_F)
  Constant6/1 -> SingleTrackModel_linear/14(c_alpha_R)
  Lenkübersetzung1/1(delta_wheel) -> Bus Selector/1  "delta_wheel"
  Bus Selector/1 -> SingleTrackModel_linear/5(SteeringAngleWheelFront [rad])  "<delta_RF>"
  BUS IN/6(delta_h) -> Lenkübersetzung1/1(delta_h)  "Steering_Angle"

== system ESM_TeslaModelS_statKreisfahrt/Timer and Bus Reset ==
  BUS_In : Inport
  Bus Creator : BusCreator  Inputs=1
  Bus Selector : BusSelector  OutputSignals=Dynamics,Drivetrain,Control Unit,Driver and Environment,Data Import  OutputAsBus=on
  Unit Delay : UnitDelay  SampleTime=-1  HasFrameUpgradeWarning=on
  BUS_Out : Outport  VectorParamsAs1DForOutWhenUnconnected=off
  wires:
  Bus Creator/1 -> BUS_Out/1  "BUS_old"
  Bus Selector/1 -> Unit Delay/1
  Unit Delay/1 -> Bus Creator/1  "Bus_Old"
  BUS_In/1 -> Bus Selector/1

== system ESM_TeslaModelS_statKreisfahrt/Control Unit/BUS IN ==
  BUS_In : Inport
  Bus Selector : BusSelector  OutputSignals=Driver and Environment.AccPedalPos [-],Driver and Environment.BrakePedalPos [-]
  BUS : Outport  VectorParamsAs1DForOutWhenUnconnected=off
  AccPedalPos [-] : Outport  Port=2  VectorParamsAs1DForOutWhenUnconnected=off
  BrakePedalPos [-] : Outport  Port=3
  wires:
  BUS_In/1 -> Bus Selector/1, BUS/1
  Bus Selector/1 -> AccPedalPos [-]/1  "<AccPedalPos [-]>"
  Bus Selector/2 -> BrakePedalPos [-]/1  "<BrakePedalPos [-]>"

== system ESM_TeslaModelS_statKreisfahrt/Control Unit/BUS OUT ==
  BUS : Inport
  In1 : Inport  Port=2
  In2 : Inport  Port=3
  In3 : Inport  Port=4
  In4 : Inport  Port=5
  Bus Creator : BusCreator  Inputs=4
  Bus Creator1 : BusCreator  Inputs=2
  Bus Selector : BusSelector  OutputSignals=Control Unit,BUS.Driver and Environment,BUS.Data Import,BUS.Bus_Old  OutputAsBus=on
  BUS_OUT : Outport  VectorParamsAs1DForOutWhenUnconnected=off
  wires:
  Bus Creator1/1 -> Bus Selector/1
  BUS/1 -> Bus Creator1/1  "BUS"
  Bus Creator/1 -> Bus Creator1/2  "Control Unit"
  Bus Selector/1 -> BUS_OUT/1
  In1/1 -> Bus Creator/1  "TargetDriveTrqFront [Nm]"
  In2/1 -> Bus Creator/2  "TargetDriveTrqRear [Nm]"
  In3/1 -> Bus Creator/3  "TargetBrakeTrqFrontAxle [Nm]"
  In4/1 -> Bus Creator/4  "TargetBrakeTrqRearAxle [Nm]"

== system ESM_TeslaModelS_statKreisfahrt/Control Unit/Control Unit Simple ==
  AccPedalPos [-] : Inport  SampleTime=LocalSampleTime
  BrakePedalPos [-] : Inport  Port=2  SampleTime=LocalSampleTime
  Abs : Abs
  Brake_Distribution_Front : Constant  Value=Brake_Distribution_Front
  Brake_Torque_Front : Product
  Brake_Torque_Rear : Product
  Constant : Constant
  Gain : Gain  Gain=-1
  MaxBrakeTorque : Constant  Value=MaxBrkTrq
  MaxMotorTorque Front : Constant  Value=MaxMotorTrqFront
  MaxMotorTorque Rear : Constant  Value=MaxMotorTrqRear
  Product : Product
  Product1 : Product
  Product2 : Product
  Subtract : Sum  Inputs=+-
  "TargetDriveTrqFront [Nm] " : Outport  SampleTime=GlobalSampleTime  VectorParamsAs1DForOutWhenUnconnected=off
  "TargetDriveTrqRear [Nm] " : Outport  Port=2
  TargetBrakeTrqFrontAxle [Nm] : Outport  Port=3  SampleTime=GlobalSampleTime  VectorParamsAs1DForOutWhenUnconnected=off
  TargetBrakeTrqRearAxle [Nm] : Outport  Port=4  SampleTime=GlobalSampleTime  VectorParamsAs1DForOutWhenUnconnected=off
  wires:
  Product/1 -> "TargetDriveTrqFront [Nm] "/1
  BrakePedalPos [-]/1 -> Product1/1
  Brake_Torque_Front/1 -> TargetBrakeTrqFrontAxle [Nm]/1
  MaxMotorTorque Front/1 -> Product/1
  Subtract/1 -> Brake_Torque_Rear/2
  Constant/1 -> Subtract/1
  AccPedalPos [-]/1 -> Product2/1, Product/2
  Brake_Torque_Rear/1 -> TargetBrakeTrqRearAxle [Nm]/1
  MaxBrakeTorque/1 -> Abs/1
  Brake_Distribution_Front/1 -> Subtract/2, Brake_Torque_Front/2
  Product1/1 -> Brake_Torque_Rear/1, Brake_Torque_Front/1
  Abs/1 -> Gain/1
  Gain/1 -> Product1/2
  MaxMotorTorque Rear/1 -> Product2/2
  Product2/1 -> "TargetDriveTrqRear [Nm] "/1

== system ESM_TeslaModelS_statKreisfahrt/Data Import/BUS IN ==
  BUS_In : Inport
  Bus Selector : BusSelector  OutputSignals=Bus_Old.Dynamics.WheelRotation/Velocity [Bus].RotationSpeedWheels.omega_F [rad/s]
  BUS : Outport  VectorParamsAs1DForOutWhenUnconnected=off
  omega_F [rad/s] : Outport  Port=2  VectorParamsAs1DForOutWhenUnconnected=off
  wires:
  BUS_In/1 -> Bus Selector/1, BUS/1
  Bus Selector/1 -> omega_F [rad/s]/1  "<omega_F [rad/s]>"

== system ESM_TeslaModelS_statKreisfahrt/Data Import/BUS OUT ==
  BUS : Inport
  In1 : Inport  Port=2
  In2 : Inport  Port=3
  In3 : Inport  Port=4
  Bus Creator : BusCreator  Inputs=3
  Bus Creator1 : BusCreator  Inputs=2
  Bus Selector : BusSelector  OutputSignals=Data Import,BUS.Bus_Old  OutputAsBus=on
  BUS_OUT : Outport  VectorParamsAs1DForOutWhenUnconnected=off
  wires:
  Bus Creator1/1 -> Bus Selector/1
  BUS/1 -> Bus Creator1/1  "BUS"
  Bus Creator/1 -> Bus Creator1/2  "Data Import"
  Bus Selector/1 -> BUS_OUT/1
  In1/1 -> Bus Creator/1  "Target_Radius [m]"
  In2/1 -> Bus Creator/2  "Traget_Velocity [m/s]"
  In3/1 -> Bus Creator/3  "Target_Steering_Angle [rad]"
